simulink model "LogicOP"  (R2020a)
settings: Solver=FixedStepDiscrete  StartTime=0.0  StopTime=10.0  RelTol=1e-3
libraries: simulink x8
settings Model: Creator=yomna  LastModifiedBy=yomna
settings OptimizationCC: DefaultParameterBehavior=Inlined  EnhancedBackFolding=on  PassReuseOutputArgsAs=Individual arguments  ZeroExternalMemoryAtStartup=off  ZeroInternalMemoryAtStartup=off  OptimizeBlockOrder=speed  DifferentSizesBufferReuse=on  OptimizationCustomize=off  EfficientTunableParamExpr=on
settings DebuggingCC: UnderspecifiedInitializationDetection=Classic  MergeDetectMultiDrivingBlocksExec=none  ParameterTunabilityLossMsg=error
settings ModelReferenceCC: PropagateSignalLabelsOutOfModel=off
settings SFSimCC: MATLABDynamicMemAlloc=off
settings RTWCC: SystemTargetFile=ert.tlc  GenCodeOnly=on  TemplateMakefile=ert_default_tmf  GenerateReport=on  IncludeHyperlinkInReport=on  LaunchReport=on  GenerateTraceInfo=on  GenerateTraceReport=on  GenerateTraceReportSl=on  GenerateTraceReportSf=on  GenerateTraceReportEml=on
settings CodeAppCC: ForceParamTrailComments=on  IgnoreCustomStorageClasses=off  OperatorAnnotations=on  SimulinkDataObjDesc=on  SFDataObjDesc=on  InsertBlockDesc=on
settings ERTTargetCC: TargetLangStandard=C99 (ISO)  GenerateSampleERTMain=on  InlinedParameterPlacement=NonHierarchical  ERTCustomFileTemplate=example_file_process.tlc

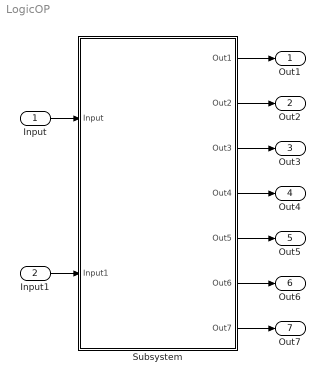
== system LogicOP ==
  Input : Inport
  Input1 : Inport  Port=2
  Subsystem : Subsystem
  Out1 : Outport
  Out2 : Outport  Port=2
  Out3 : Outport  Port=3
  Out4 : Outport  Port=4
  Out5 : Outport  Port=5
  Out6 : Outport  Port=6
  Out7 : Outport  Port=7
  wires:
  Input/1 -> Subsystem/1(Input)
  Input1/1 -> Subsystem/2(Input1)
  Subsystem/2(Out2) -> Out2/1
  Subsystem/7(Out7) -> Out7/1
  Subsystem/6(Out6) -> Out6/1
  Subsystem/4(Out4) -> Out4/1
  Subsystem/5(Out5) -> Out5/1
  Subsystem/3(Out3) -> Out3/1
  Subsystem/1(Out1) -> Out1/1

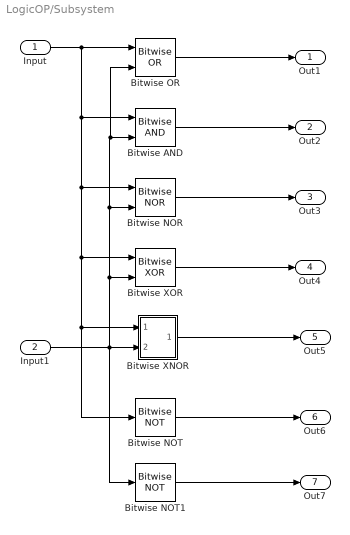
== system LogicOP/Subsystem ==
  Input : Inport  OutDataTypeStr=uint8
  Input1 : Inport  Port=2  OutDataTypeStr=uint8
  Bitwise AND : simulink/Logic and Bit Operations/Bitwise Operator  logicop=AND  UseBitMask=off  NumInputPorts=2  BitMask=bin2dec('11011001')  BitMaskRealWorld=Stored Integer
  Bitwise NOR : simulink/Logic and Bit Operations/Bitwise Operator  logicop=NOR  UseBitMask=off  NumInputPorts=2  BitMask=bin2dec('11011001')  BitMaskRealWorld=Stored Integer
  Bitwise NOT : simulink/Logic and Bit Operations/Bitwise Operator  logicop=NOT  UseBitMask=off  BitMask=bin2dec('11011001')  BitMaskRealWorld=Stored Integer
  Bitwise NOT1 : simulink/Logic and Bit Operations/Bitwise Operator  logicop=NOT  UseBitMask=off  BitMask=bin2dec('11011001')  BitMaskRealWorld=Stored Integer
  Bitwise OR : simulink/Logic and Bit Operations/Bitwise Operator  logicop=OR  UseBitMask=off  NumInputPorts=2  BitMask=bin2dec('11011001')  BitMaskRealWorld=Stored Integer
  Bitwise XNOR : Subsystem
  Bitwise XOR : simulink/Logic and Bit Operations/Bitwise Operator  logicop=XOR  UseBitMask=off  NumInputPorts=2  BitMask=bin2dec('11011001')  BitMaskRealWorld=Stored Integer
  Out1 : Outport
  Out2 : Outport  Port=2
  Out3 : Outport  Port=3
  Out4 : Outport  Port=4
  Out5 : Outport  Port=5
  Out6 : Outport  Port=6
  Out7 : Outport  Port=7
  wires:
  Bitwise NOT/1 -> Out6/1
  Bitwise AND/1 -> Out2/1
  Input1/1 -> Bitwise NOT1/1, Bitwise XNOR/2(In2), Bitwise OR/2, Bitwise AND/2, Bitwise NOR/2, Bitwise XOR/2
  Input/1 -> Bitwise NOT/1, Bitwise XNOR/1(In1), Bitwise XOR/1, Bitwise NOR/1, Bitwise AND/1, Bitwise OR/1
  Bitwise OR/1 -> Out1/1
  Bitwise XOR/1 -> Out4/1
  Bitwise NOR/1 -> Out3/1
  Bitwise XNOR/1(Out1) -> Out5/1
  Bitwise NOT1/1 -> Out7/1

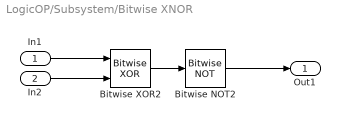
== system LogicOP/Subsystem/Bitwise XNOR ==
  In1 : Inport
  In2 : Inport  Port=2
  Bitwise NOT2 : simulink/Logic and Bit Operations/Bitwise Operator  logicop=NOT  UseBitMask=off  BitMask=bin2dec('11011001')  BitMaskRealWorld=Stored Integer
  Bitwise XOR2 : simulink/Logic and Bit Operations/Bitwise Operator  logicop=XOR  UseBitMask=off  NumInputPorts=2  BitMask=bin2dec('11011001')  BitMaskRealWorld=Stored Integer
  Out1 : Outport
  wires:
  Bitwise XOR2/1 -> Bitwise NOT2/1
  Bitwise NOT2/1 -> Out1/1
  In2/1 -> Bitwise XOR2/2
  In1/1 -> Bitwise XOR2/1
